simulink model "ReadGagesLong"  (R2019a)
settings: Solver=ode4  StartTime=0.0  StopTime=9999999  FixedStep=0.01  RelTol=1e-3
model workspace (MAT data in the model file):
  myVar = 5.12
undefined symbols (not defined in the file or in its folder): Advantech, PCI
libraries: sldrtlib x12
settings Model: SimulationMode=external  ExtModeTrigDuration=10000  ExtModeArchiveMode=auto  ExtModeArchiveFileName=gages_simout  ExtModeArchiveDirName=G:\Mi unidad\ROBOESPAS_COLABORATIVE\RoboespasMatlab\Develop\Common\FTSensor_Tmp  Creator=SyS  LastModifiedBy=roboespas
settings DataIOCC: MaxDataPoints=10000  SaveFinalState=on  SaveFormat=Array  SignalLoggingSaveFormat=ModelDataLogs  ReturnWorkspaceOutputs=off
settings OptimizationCC: BlockReduction=off  BooleanDataType=off  ExpressionDepthLimit=2147483647  InitFltsAndDblsToZero=on
settings DebuggingCC: SaveWithParameterizedLinksMsg=none  UnderspecifiedInitializationDetection=Classic  MergeDetectMultiDrivingBlocksExec=none  SignalResolutionControl=TryResolveAllWithWarning  MultiTaskDSMMsg=warning  MultiTaskCondExecSysMsg=none  FcnCallInpInsideContextMsg=warning  StateNameClashWarn=warning  SFUnexpectedBacktrackingDiag=warning  SFNoUnconditionalDefaultTransitionDiag=warning  SFExecutionAtInitializationDiag=none  ArithmeticOperatorsInVariantConditions=warning
settings ModelReferenceCC: PropagateSignalLabelsOutOfModel=off
settings RTWCC: SystemTargetFile=sldrt.tlc  TemplateMakefile=sldrt.tmf  Description=Simulink Desktop Real-Time  RTWCompilerOptimization=on
settings CodeAppCC: MaxIdLength=95  StateflowObjectComments=on
settings SimulinkDesktopRealTimeCC: TargetPreCompLibLocation=C:\Program Files\MATLAB\R2019a\toolbox\sldrt\lib\win64  TargetLangStandard=C89/C90 (ANSI)  ModelReferenceCompliant=off  CompOptLevelCompliant=off  SupportVariableSizeSignals=off  PreserveStateflowLocalDataDimensions=off
settings ConfigComp: CovMetricSettings=dw  CovHtmlReporting=on  CovSaveCumulativeToWorkspaceVar=on  CovSaveSingleToWorkspaceVar=on

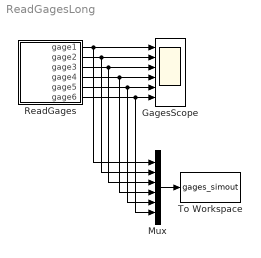
== system ReadGagesLong ==
  GagesScope : Scope  NumInputPorts=6
  Mux : Mux  Inputs=6
  "ReadGages " : Subsystem
  To Workspace : ToWorkspace  VariableName=gages_simout  SaveFormat=Structure With Time  SampleTime=-1
  wires:
  "ReadGages "/6(gage6) -> GagesScope/6, Mux/6
  "ReadGages "/2(gage2) -> GagesScope/2, Mux/2
  "ReadGages "/5(gage5) -> GagesScope/5, Mux/5
  "ReadGages "/1(gage1) -> GagesScope/1, Mux/1
  "ReadGages "/3(gage3) -> GagesScope/3, Mux/3
  "ReadGages "/4(gage4) -> GagesScope/4, Mux/4
  Mux/1 -> To Workspace/1

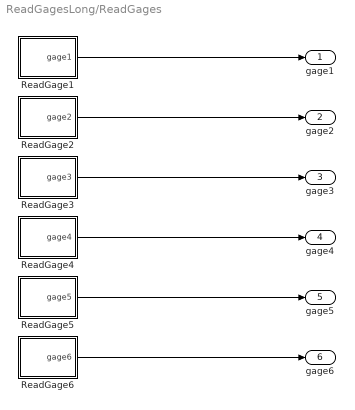
== system ReadGagesLong/ReadGages  ==
  ReadGage1 : Subsystem
  ReadGage2 : Subsystem
  ReadGage3 : Subsystem
  ReadGage4 : Subsystem
  ReadGage5 : Subsystem
  ReadGage6 : Subsystem
  gage1 : Outport
  gage2 : Outport  Port=2
  gage3 : Outport  Port=3
  gage4 : Outport  Port=4
  gage5 : Outport  Port=5
  gage6 : Outport  Port=6
  wires:
  ReadGage1/1(gage1) -> gage1/1
  ReadGage2/1(gage2) -> gage2/1
  ReadGage3/1(gage3) -> gage3/1
  ReadGage4/1(gage4) -> gage4/1
  ReadGage5/1("gage5 ") -> gage5/1
  ReadGage6/1(gage6) -> gage6/1

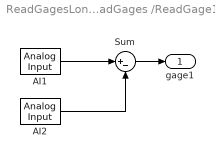
== system ReadGagesLong/ReadGages /ReadGage1 ==
  AI1 : sldrtlib/Analog Input  SampleTime=0.01  MaxMissedTicks=10  ShowMissedTicks=off  YieldWhenWaiting=off  DrvName=Advantech/PCI-1711  DrvAddress=4294967295  DrvOptions=zeros(1,0)  Channels=1  RangeMode=1  VoltRange=1  DataType=1
      settings: AttributesFormatString=Advantech\nPCI-1711 [auto]  SourceProductName=Simulink Desktop Real-Time
  AI2 : sldrtlib/Analog Input  SampleTime=0.01  MaxMissedTicks=10  ShowMissedTicks=off  YieldWhenWaiting=off  DrvName=Advantech/PCI-1711  DrvAddress=4294967295  DrvOptions=zeros(1,0)  Channels=2  RangeMode=1  VoltRange=1  DataType=1
      settings: AttributesFormatString=Advantech\nPCI-1711 [auto]  SourceProductName=Simulink Desktop Real-Time
  Sum : Sum  Inputs=|+-
  gage1 : Outport
  wires:
  AI1/1 -> Sum/1
  AI2/1 -> Sum/2
  Sum/1 -> gage1/1

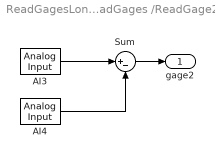
== system ReadGagesLong/ReadGages /ReadGage2 ==
  AI3 : sldrtlib/Analog Input  SampleTime=0.01  MaxMissedTicks=10  ShowMissedTicks=off  YieldWhenWaiting=off  DrvName=Advantech/PCI-1711  DrvAddress=4294967295  DrvOptions=zeros(1,0)  Channels=3  RangeMode=1  VoltRange=1  DataType=1
      settings: AttributesFormatString=Advantech\nPCI-1711 [auto]  SourceProductName=Simulink Desktop Real-Time
  AI4 : sldrtlib/Analog Input  SampleTime=0.01  MaxMissedTicks=10  ShowMissedTicks=off  YieldWhenWaiting=off  DrvName=Advantech/PCI-1711  DrvAddress=4294967295  DrvOptions=zeros(1,0)  Channels=4  RangeMode=1  VoltRange=1  DataType=1
      settings: AttributesFormatString=Advantech\nPCI-1711 [auto]  SourceProductName=Simulink Desktop Real-Time
  Sum : Sum  Inputs=|+-
  gage2 : Outport
  wires:
  AI3/1 -> Sum/1
  AI4/1 -> Sum/2
  Sum/1 -> gage2/1

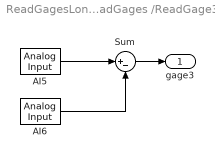
== system ReadGagesLong/ReadGages /ReadGage3 ==
  AI5 : sldrtlib/Analog Input  SampleTime=0.01  MaxMissedTicks=10  ShowMissedTicks=off  YieldWhenWaiting=off  DrvName=Advantech/PCI-1711  DrvAddress=4294967295  DrvOptions=zeros(1,0)  Channels=5  RangeMode=1  VoltRange=1  DataType=1
      settings: AttributesFormatString=Advantech\nPCI-1711 [auto]  SourceProductName=Simulink Desktop Real-Time
  AI6 : sldrtlib/Analog Input  SampleTime=0.01  MaxMissedTicks=10  ShowMissedTicks=off  YieldWhenWaiting=off  DrvName=Advantech/PCI-1711  DrvAddress=4294967295  DrvOptions=zeros(1,0)  Channels=6  RangeMode=1  VoltRange=1  DataType=1
      settings: AttributesFormatString=Advantech\nPCI-1711 [auto]  SourceProductName=Simulink Desktop Real-Time
  Sum : Sum  Inputs=|+-
  gage3 : Outport
  wires:
  AI5/1 -> Sum/1
  AI6/1 -> Sum/2
  Sum/1 -> gage3/1

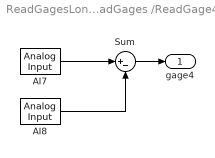
== system ReadGagesLong/ReadGages /ReadGage4 ==
  AI7 : sldrtlib/Analog Input  SampleTime=0.01  MaxMissedTicks=10  ShowMissedTicks=off  YieldWhenWaiting=off  DrvName=Advantech/PCI-1711  DrvAddress=4294967295  DrvOptions=zeros(1,0)  Channels=7  RangeMode=1  VoltRange=1  DataType=1
      settings: AttributesFormatString=Advantech\nPCI-1711 [auto]  SourceProductName=Simulink Desktop Real-Time
  AI8 : sldrtlib/Analog Input  SampleTime=0.01  MaxMissedTicks=10  ShowMissedTicks=off  YieldWhenWaiting=off  DrvName=Advantech/PCI-1711  DrvAddress=4294967295  DrvOptions=zeros(1,0)  Channels=8  RangeMode=1  VoltRange=1  DataType=1
      settings: AttributesFormatString=Advantech\nPCI-1711 [auto]  SourceProductName=Simulink Desktop Real-Time
  Sum : Sum  Inputs=|+-
  gage4 : Outport
  wires:
  AI7/1 -> Sum/1
  AI8/1 -> Sum/2
  Sum/1 -> gage4/1

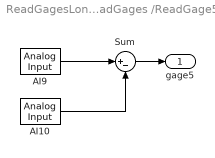
== system ReadGagesLong/ReadGages /ReadGage5 ==
  AI10 : sldrtlib/Analog Input  SampleTime=0.01  MaxMissedTicks=10  ShowMissedTicks=off  YieldWhenWaiting=off  DrvName=Advantech/PCI-1711  DrvAddress=4294967295  DrvOptions=zeros(1,0)  Channels=10  RangeMode=1  VoltRange=1  DataType=1
      settings: AttributesFormatString=Advantech\nPCI-1711 [auto]  SourceProductName=Simulink Desktop Real-Time
  AI9 : sldrtlib/Analog Input  SampleTime=0.01  MaxMissedTicks=10  ShowMissedTicks=off  YieldWhenWaiting=off  DrvName=Advantech/PCI-1711  DrvAddress=4294967295  DrvOptions=zeros(1,0)  Channels=9  RangeMode=1  VoltRange=1  DataType=1
      settings: AttributesFormatString=Advantech\nPCI-1711 [auto]  SourceProductName=Simulink Desktop Real-Time
  Sum : Sum  Inputs=|+-
  "gage5 " : Outport
  wires:
  AI9/1 -> Sum/1
  AI10/1 -> Sum/2
  Sum/1 -> "gage5 "/1

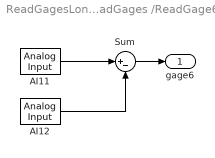
== system ReadGagesLong/ReadGages /ReadGage6 ==
  AI11 : sldrtlib/Analog Input  SampleTime=0.01  MaxMissedTicks=10  ShowMissedTicks=off  YieldWhenWaiting=off  DrvName=Advantech/PCI-1711  DrvAddress=4294967295  DrvOptions=zeros(1,0)  Channels=11  RangeMode=1  VoltRange=1  DataType=1
      settings: AttributesFormatString=Advantech\nPCI-1711 [auto]  SourceProductName=Simulink Desktop Real-Time
  AI12 : sldrtlib/Analog Input  SampleTime=0.01  MaxMissedTicks=10  ShowMissedTicks=off  YieldWhenWaiting=off  DrvName=Advantech/PCI-1711  DrvAddress=4294967295  DrvOptions=zeros(1,0)  Channels=12  RangeMode=1  VoltRange=1  DataType=1
      settings: AttributesFormatString=Advantech\nPCI-1711 [auto]  SourceProductName=Simulink Desktop Real-Time
  Sum : Sum  Inputs=|+-
  gage6 : Outport
  wires:
  AI11/1 -> Sum/1
  AI12/1 -> Sum/2
  Sum/1 -> gage6/1
